simulink model "Liquid_Level_Control_Continuous_1_24_RoaaTareq"  (R2022a)
settings: Solver=VariableStepAuto  StartTime=0.0  StopTime=15  RelTol=1e-3
settings Model: Creator=hp  LastModifiedBy=hp

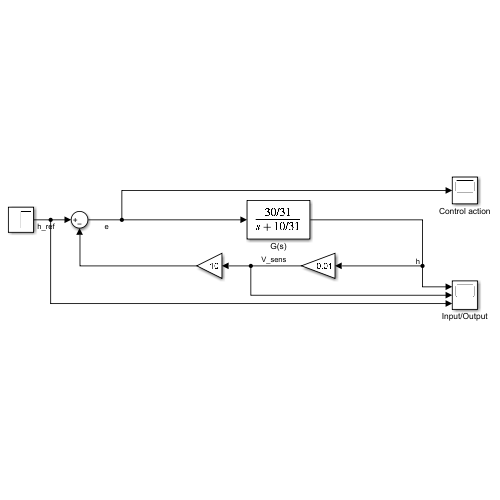
[thumbnail: Simulink's stored preview of the top-level diagram]
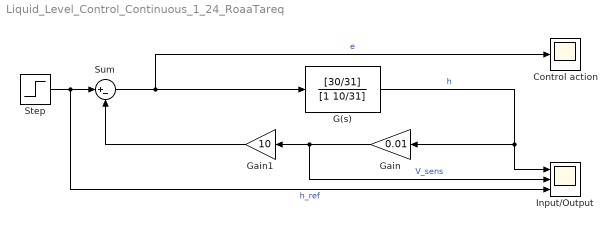
== system Liquid_Level_Control_Continuous_1_24_RoaaTareq ==
  Control action : Scope
  G(s) : TransferFcn  Numerator=[30/31]  Denominator=[1 10/31]
  Gain : Gain  Gain=0.01
  Gain1 : Gain  Gain=10
  Input/Output : Scope  NumInputPorts=3
  Step : Step  Time=0  After=10  SampleTime=0
  Sum : Sum  Inputs=|+-
  wires:
  G(s)/1 -> Input/Output/1, Gain/1  "h"
  Gain1/1 -> Sum/2
  Step/1 -> Input/Output/3, Sum/1  "h_ref"
  Sum/1 -> G(s)/1, Control action/1  "e"
  Gain/1 -> Gain1/1, Input/Output/2  "V_sens"
